simulink model "Linmod_XY_axis_PID_cascade_2021_state_estimator_extra_values"  (R2022b)
settings: Solver=ode4  StartTime=0.0  StopTime=68  FixedStep=1/400  RelTol=1e-3
undefined symbols (not defined in the file): Quad
libraries: simulink x2
settings Model: Creator=laurentburlion  LastModifiedBy=blank
settings ModelReferenceCC: EnableRefExpFcnMdlSchedulingChecks=on

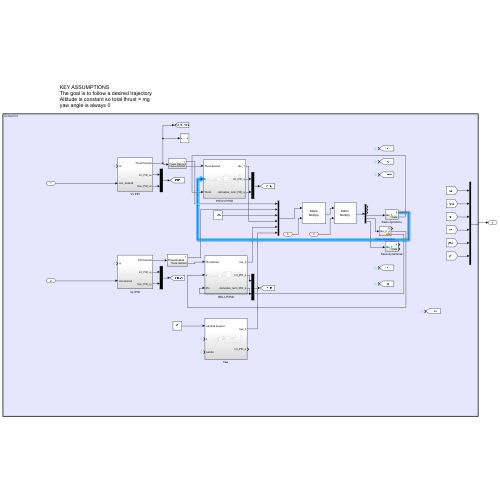
[thumbnail: Simulink's stored preview of the top-level diagram]
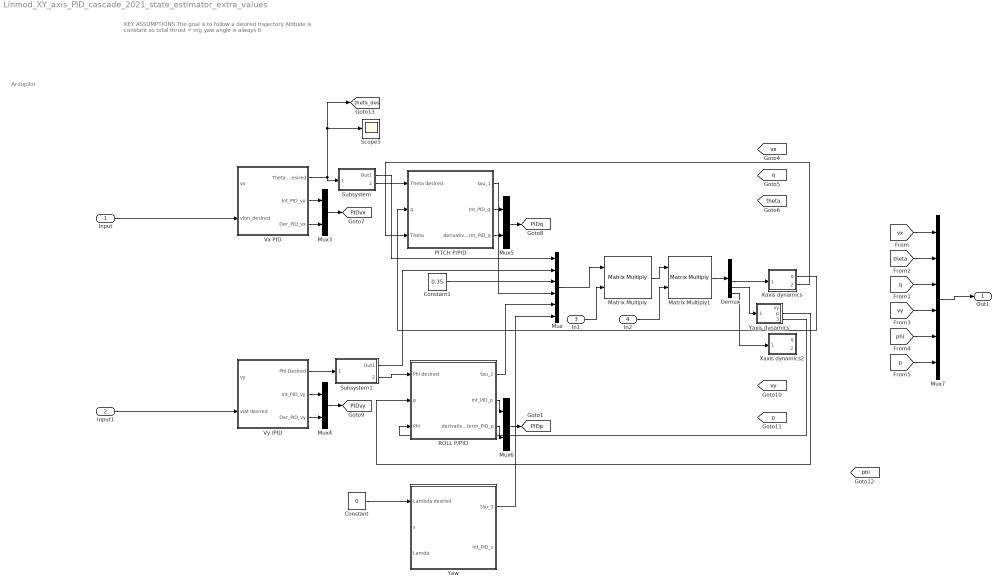
== system Linmod_XY_axis_PID_cascade_2021_state_estimator_extra_values ==
  note: Ardupilot
  note: KEY ASSUMPTIONS
      | The goal is to follow a desired trajectory
      | Altitude is constant so total thrust = mg
      | yaw angle is always 0
  Input : Inport
  Input1 : Inport  Port=2
  In1 : Inport  Port=3
  In2 : Inport  Port=4
  Constant : Constant  Value=0
  Constant1 : Constant  Value=0.35
  Demux : Demux  Outputs=6
  Matrix Multiply : Product  Multiplication=Matrix(*)
  Matrix Multiply1 : Product  Multiplication=Matrix(*)
  Mux : Mux  Inputs=6
  Mux{3..6} (4 alike) : Mux  Inputs=2
  Mux7 : Mux  Inputs=6
  PITCH P/PID : Subsystem
  ROLL P/PID : Subsystem
  Scope5 : Scope
  Subsystem : Subsystem
  Subsystem1 : Subsystem
  Vx PID : Subsystem
  Vy /PID : Subsystem
  Xaxis dynamics : Subsystem
  Xaxis dynamics2 : Subsystem
  "Yaw " : Subsystem
  Yaxis dynamics : Subsystem
  Out1 : Outport
  tag scope: PIDp=global, PIDq=global, PIDvx=global, PIDvy=global, p=global, phi=global, q=global, theta=global, theta_des=global, vx=global, vy=global
  wires:
  Vy /PID/1(Phi Desired) -> Subsystem1/1(Theta Desired)
  Vx PID/1(Theta Desired) -> Subsystem/1(Theta Desired), [theta_des], Scope5/1
  Vy /PID/3(Der_PID_vy) -> Mux4/2
  Vy /PID/2(Int_PID_vy) -> Mux4/1
  Mux4/1 -> [PIDvy]
  Vx PID/2(Int_PID_vx) -> Mux3/1
  Vx PID/3(Der_PID_vx) -> Mux3/2
  Mux3/1 -> [PIDvx]
  PITCH P/PID/3(derivative_term_PID_q) -> Mux5/2
  PITCH P/PID/2(Int_PID_q) -> Mux5/1
  Mux5/1 -> [PIDq]
  ROLL P/PID/2(Int_PID_p) -> Mux6/1
  ROLL P/PID/3(derivative_term_PID_p) -> Mux6/2
  Mux6/1 -> [PIDp]
  Input/1 -> Vx PID/2(vlon_desired)
  Input1/1 -> Vy /PID/2(vlat desired)
  [vx] -> Mux7/1
  [q] -> Mux7/3
  [theta] -> Mux7/2
  [vy] -> Mux7/4
  [p] -> Mux7/6
  [phi] -> Mux7/5
  Mux7/1 -> Out1/1
  Subsystem/2(Theta desired) -> PITCH P/PID/1(Theta desired)
  Subsystem1/2(Theta desired) -> ROLL P/PID/1(Phi desired)
  Constant/1 -> "Yaw "/1(Lambda desired)
  Subsystem/1(Out1) -> Mux/1
  Subsystem1/1(Out1) -> Mux/2
  PITCH P/PID/1(tau_1) -> Mux/4
  ROLL P/PID/1(tau_2) -> Mux/5
  "Yaw "/1(tau_3) -> Mux/6
  Mux/1 -> Matrix Multiply/1
  Constant1/1 -> Mux/3
  In1/1 -> Matrix Multiply/2
  Matrix Multiply/1 -> Matrix Multiply1/1
  In2/1 -> Matrix Multiply1/2
  Matrix Multiply1/1 -> Demux/1
  Demux/4 -> Xaxis dynamics/1(tau_1)
  Demux/5 -> Yaxis dynamics/1(tau_2)
  Demux/6 -> Xaxis dynamics2/1(tau_1)
  Xaxis dynamics/1(q) -> PITCH P/PID/2(q)
  Xaxis dynamics/2(theta) -> PITCH P/PID/3(Theta)
  Yaxis dynamics/2(p) -> ROLL P/PID/2(p)
  Yaxis dynamics/3(phi) -> ROLL P/PID/3(Phi)

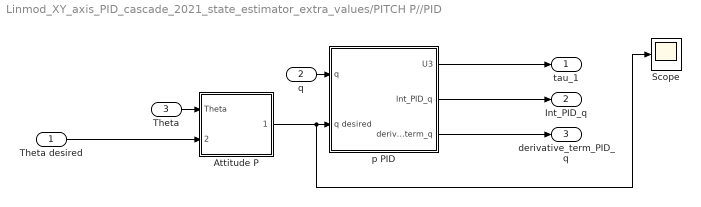
== system Linmod_XY_axis_PID_cascade_2021_state_estimator_extra_values/PITCH P//PID ==
  Theta desired : Inport
  q : Inport  Port=2
  Theta : Inport  Port=3
  Attitude P : Subsystem
  Scope : Scope
  p PID : Subsystem
  tau_1 : Outport
  Int_PID_q : Outport  Port=2
  derivative_term_PID_q : Outport  Port=3
  wires:
  p PID/1(U3) -> tau_1/1
  Attitude P/1(q desired) -> Scope/1, p PID/2(q desired)
  Theta/1 -> Attitude P/1(Theta)
  q/1 -> p PID/1(q)
  Theta desired/1 -> Attitude P/2(Theta desired)
  p PID/2(Int_PID_q) -> Int_PID_q/1
  p PID/3(derivative_term_q) -> derivative_term_PID_q/1

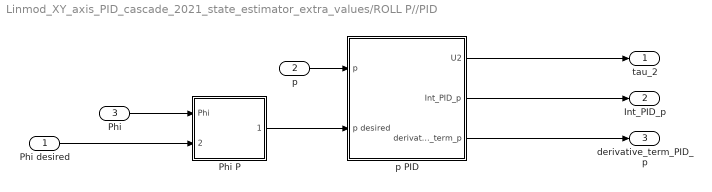
== system Linmod_XY_axis_PID_cascade_2021_state_estimator_extra_values/ROLL P//PID ==
  Phi desired : Inport
  p : Inport  Port=2
  Phi : Inport  Port=3
  Phi P : Subsystem
  p PID : Subsystem
  tau_2 : Outport
  Int_PID_p : Outport  Port=2
  derivative_term_PID_p : Outport  Port=3
  wires:
  Phi desired/1 -> Phi P/2(Phi desired)
  p/1 -> p PID/1(p)
  Phi/1 -> Phi P/1(Phi)
  Phi P/1(p desired) -> p PID/2(p desired)
  p PID/1(U2) -> tau_2/1
  p PID/2(Int_PID_p) -> Int_PID_p/1
  p PID/3(derivative_term_p) -> derivative_term_PID_p/1

== system Linmod_XY_axis_PID_cascade_2021_state_estimator_extra_values/Subsystem ==
  Theta Desired : Inport
  Constant : Constant  Value=0.0
  Sine : simulink/Lookup Tables/Sine  Formula=sin(2*pi*u)  NumDataPoints=(2^5)+1  OutputWordLength=16  InternalRulePriority=Speed
  Out1 : Outport
  Theta desired : Outport  Port=2
  wires:
  Theta Desired/1 -> Sine/1
  Sine/1 -> Out1/1
  Constant/1 -> Theta desired/1

== system Linmod_XY_axis_PID_cascade_2021_state_estimator_extra_values/Subsystem1 ==
  Theta Desired : Inport
  Constant : Constant  Value=0.0
  Cosine : simulink/Lookup Tables/Cosine  Formula=cos(2*pi*u)  NumDataPoints=(2^5)+1  OutputWordLength=16  InternalRulePriority=Speed
  Out1 : Outport
  Theta desired : Outport  Port=2
  wires:
  Theta Desired/1 -> Cosine/1
  Cosine/1 -> Out1/1
  Constant/1 -> Theta desired/1

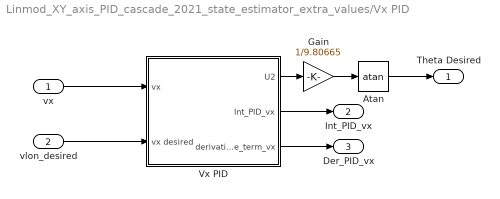
== system Linmod_XY_axis_PID_cascade_2021_state_estimator_extra_values/Vx PID ==
  vx : Inport
  vlon_desired : Inport  Port=2
  Atan : Trigonometry  Operator=atan
  Gain : Gain  Gain=1/9.80665
  Vx PID : Subsystem
  Theta Desired : Outport
  Int_PID_vx : Outport  Port=2
  Der_PID_vx : Outport  Port=3
  wires:
  vlon_desired/1 -> Vx PID/2(vx desired)
  vx/1 -> Vx PID/1(vx)
  Vx PID/2(Int_PID_vx) -> Int_PID_vx/1
  Vx PID/3(derivative_term_vx) -> Der_PID_vx/1
  Vx PID/1(U2) -> Gain/1
  Gain/1 -> Atan/1
  Atan/1 -> Theta Desired/1

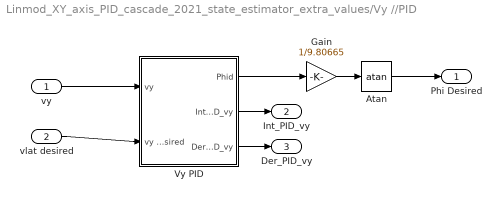
== system Linmod_XY_axis_PID_cascade_2021_state_estimator_extra_values/Vy //PID ==
  vy : Inport
  vlat desired : Inport  Port=2
  Atan : Trigonometry  Operator=atan
  Gain : Gain  Gain=1/9.80665
  Vy PID : Subsystem
  Phi Desired : Outport
  Int_PID_vy : Outport  Port=2
  Der_PID_vy : Outport  Port=3
  wires:
  Vy PID/2(Int_PID_vy) -> Int_PID_vy/1
  vy/1 -> Vy PID/1(vy)
  vlat desired/1 -> Vy PID/2(vy desired)
  Vy PID/3(Derivative_PID_vy) -> Der_PID_vy/1
  Vy PID/1(Phid) -> Gain/1
  Gain/1 -> Atan/1
  Atan/1 -> Phi Desired/1

== system Linmod_XY_axis_PID_cascade_2021_state_estimator_extra_values/Xaxis dynamics ==
  tau_1 : Inport
  Gain : Gain  Gain=1/Quad.Jy
  Integrator : Integrator
  Integrator1 : Integrator
  Scope : Scope
  q : Outport
  theta : Outport  Port=2
  wires:
  Integrator1/1 -> Scope/1, theta/1
  Integrator/1 -> q/1, Integrator1/1
  Gain/1 -> Integrator/1
  tau_1/1 -> Gain/1

== system Linmod_XY_axis_PID_cascade_2021_state_estimator_extra_values/Xaxis dynamics2 ==
  tau_1 : Inport
  Gain : Gain  Gain=1/Quad.Jy
  Integrator : Integrator
  Integrator1 : Integrator
  Scope : Scope
  q : Outport
  theta : Outport  Port=2
  wires:
  Integrator1/1 -> Scope/1, theta/1
  Integrator/1 -> q/1, Integrator1/1
  Gain/1 -> Integrator/1
  tau_1/1 -> Gain/1

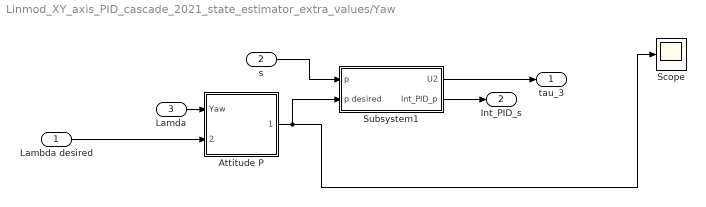
== system Linmod_XY_axis_PID_cascade_2021_state_estimator_extra_values/Yaw  ==
  Lambda desired : Inport
  s : Inport  Port=2
  "Lamda " : Inport  Port=3
  Attitude P : Subsystem
  Scope : Scope
  Subsystem1 : Subsystem
  tau_3 : Outport
  Int_PID_s : Outport  Port=2
  wires:
  s/1 -> Subsystem1/1(p)
  Subsystem1/1(U2) -> tau_3/1
  Subsystem1/2(Int_PID_p) -> Int_PID_s/1
  Attitude P/1(q desired) -> Subsystem1/2(p desired), Scope/1
  Lambda desired/1 -> Attitude P/2(Yaw desired)
  "Lamda "/1 -> Attitude P/1(Yaw)

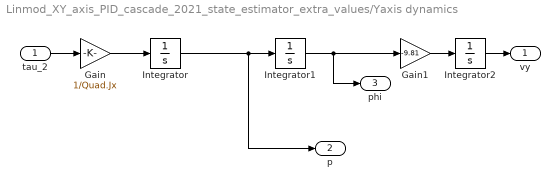
== system Linmod_XY_axis_PID_cascade_2021_state_estimator_extra_values/Yaxis dynamics ==
  tau_2 : Inport
  Gain : Gain  Gain=1/Quad.Jx
  Gain1 : Gain  Gain=-9.81
  Integrator : Integrator
  Integrator1 : Integrator
  Integrator2 : Integrator
  vy : Outport
  p : Outport  Port=2
  phi : Outport  Port=3
  wires:
  tau_2/1 -> Gain/1
  Gain/1 -> Integrator/1
  Integrator/1 -> Integrator1/1, p/1
  Integrator1/1 -> phi/1, Gain1/1
  Gain1/1 -> Integrator2/1
  Integrator2/1 -> vy/1

== system Linmod_XY_axis_PID_cascade_2021_state_estimator_extra_values/PITCH P//PID/Attitude P ==
  Theta : Inport
  Theta desired : Inport  Port=2
  Kp : Gain  Gain=Quad.phi_KP
  Theta Error : Sum  Inputs=+-
  q desired : Outport
  wires:
  Theta Error/1 -> Kp/1
  Kp/1 -> q desired/1
  Theta desired/1 -> Theta Error/1
  Theta/1 -> Theta Error/2

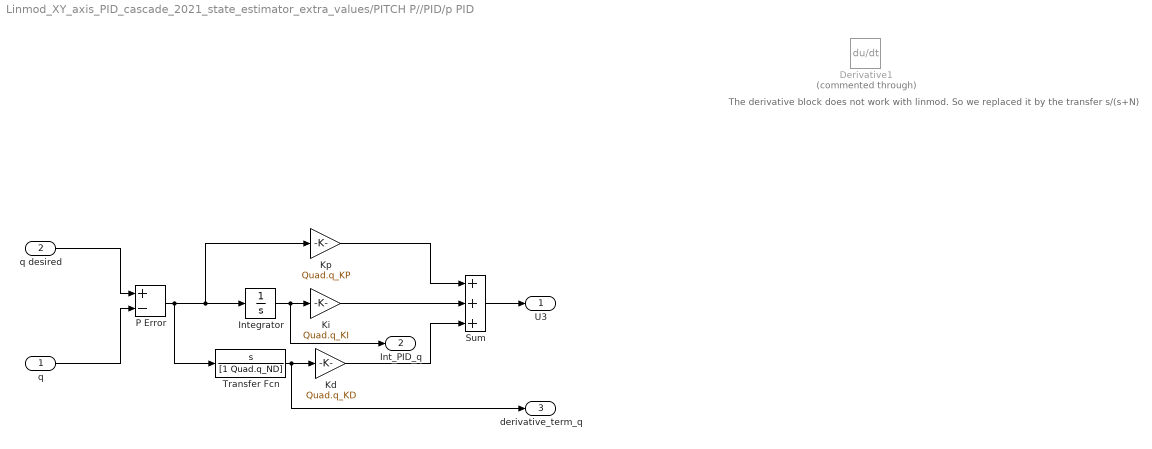
== system Linmod_XY_axis_PID_cascade_2021_state_estimator_extra_values/PITCH P//PID/p PID ==
  note: The derivative block does not work with linmod. So we replaced it by the transfer s/(s+N)
  q : Inport
  q desired : Inport  Port=2
  Derivative1 : Derivative  Commented=through
  Integrator : Integrator
  Kd : Gain  Gain=Quad.q_KD
  Ki : Gain  Gain=Quad.q_KI
  Kp : Gain  Gain=Quad.q_KP
  P Error : Sum  Inputs=+-
  Sum : Sum  Inputs=+++
  Transfer Fcn : TransferFcn  Numerator=[1 0]  Denominator=[1 Quad.q_ND]
  U3 : Outport
  Int_PID_q : Outport  Port=2
  derivative_term_q : Outport  Port=3
  wires:
  Ki/1 -> Sum/2
  Kd/1 -> Sum/3
  Integrator/1 -> Int_PID_q/1, Ki/1
  Sum/1 -> U3/1
  Kp/1 -> Sum/1
  q desired/1 -> P Error/1
  q/1 -> P Error/2
  P Error/1 -> Transfer Fcn/1, Kp/1, Integrator/1
  Transfer Fcn/1 -> derivative_term_q/1, Kd/1

== system Linmod_XY_axis_PID_cascade_2021_state_estimator_extra_values/ROLL P//PID/Phi P ==
  Phi : Inport
  Phi desired : Inport  Port=2
  Kp : Gain  Gain=Quad.phi_KP
  Phi Error : Sum  Inputs=+-
  p desired : Outport
  wires:
  Phi/1 -> Phi Error/2
  Phi desired/1 -> Phi Error/1
  Kp/1 -> p desired/1
  Phi Error/1 -> Kp/1

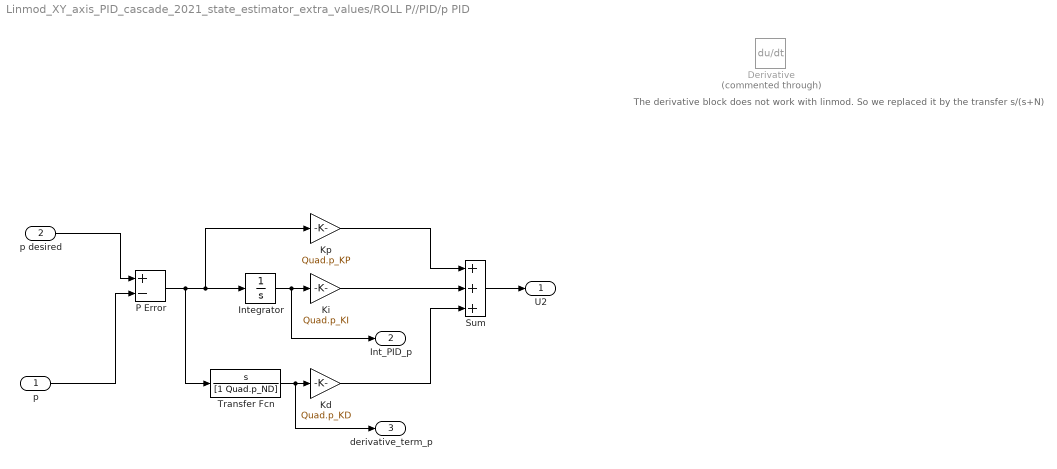
== system Linmod_XY_axis_PID_cascade_2021_state_estimator_extra_values/ROLL P//PID/p PID ==
  note: The derivative block does not work with linmod. So we replaced it by the transfer s/(s+N)
  p : Inport
  p desired : Inport  Port=2
  Derivative : Derivative  Commented=through
  Integrator : Integrator
  Kd : Gain  Gain=Quad.p_KD
  Ki : Gain  Gain=Quad.p_KI
  Kp : Gain  Gain=Quad.p_KP
  P Error : Sum  Inputs=+-
  Sum : Sum  Inputs=+++
  Transfer Fcn : TransferFcn  Numerator=[1 0]  Denominator=[1 Quad.p_ND]
  U2 : Outport
  Int_PID_p : Outport  Port=2
  derivative_term_p : Outport  Port=3
  wires:
  p/1 -> P Error/2
  p desired/1 -> P Error/1
  Kp/1 -> Sum/1
  Sum/1 -> U2/1
  Integrator/1 -> Int_PID_p/1, Ki/1
  Kd/1 -> Sum/3
  Ki/1 -> Sum/2
  P Error/1 -> Transfer Fcn/1, Integrator/1, Kp/1
  Transfer Fcn/1 -> derivative_term_p/1, Kd/1

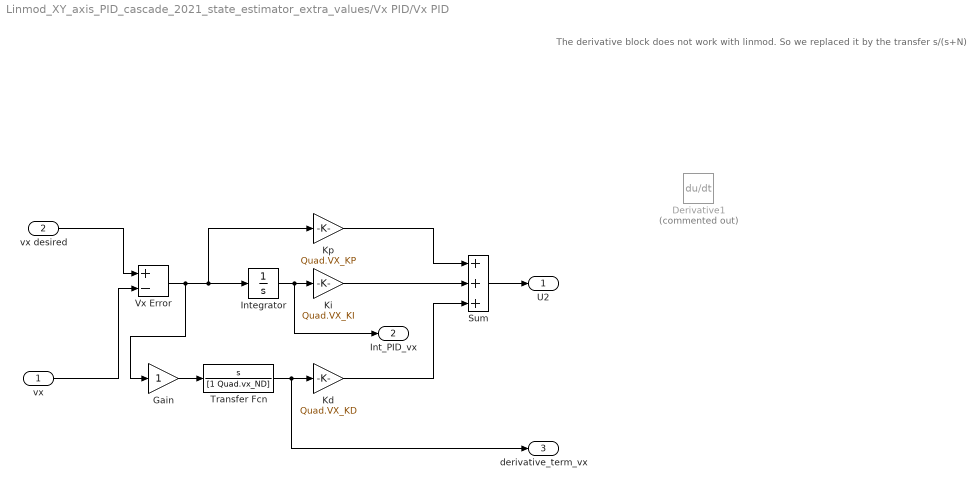
== system Linmod_XY_axis_PID_cascade_2021_state_estimator_extra_values/Vx PID/Vx PID ==
  note: The derivative block does not work with linmod. So we replaced it by the transfer s/(s+N)
  vx : Inport
  vx desired : Inport  Port=2
  Derivative1 : Derivative  Commented=on
  Gain : Gain
  Integrator : Integrator
  Kd : Gain  Gain=Quad.VX_KD
  Ki : Gain  Gain=Quad.VX_KI
  Kp : Gain  Gain=Quad.VX_KP
  Sum : Sum  Inputs=+++
  Transfer Fcn : TransferFcn  Numerator=[1 0]  Denominator=[1 Quad.vx_ND]
  Vx Error : Sum  Inputs=+-
  U2 : Outport
  Int_PID_vx : Outport  Port=2
  derivative_term_vx : Outport  Port=3
  wires:
  vx/1 -> Vx Error/2
  vx desired/1 -> Vx Error/1
  Kp/1 -> Sum/1
  Sum/1 -> U2/1
  Vx Error/1 -> Gain/1, Integrator/1, Kp/1
  Integrator/1 -> Int_PID_vx/1, Ki/1
  Kd/1 -> Sum/3
  Gain/1 -> Transfer Fcn/1
  Ki/1 -> Sum/2
  Transfer Fcn/1 -> derivative_term_vx/1, Kd/1

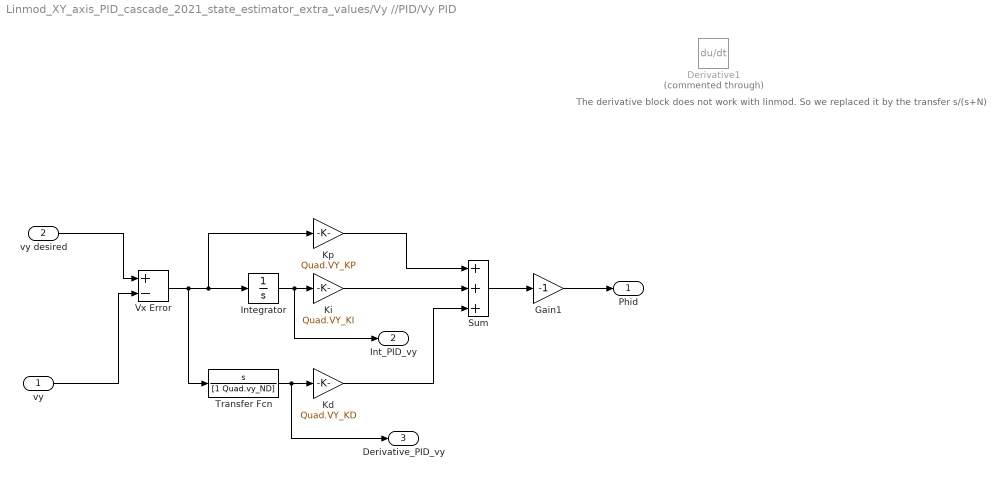
== system Linmod_XY_axis_PID_cascade_2021_state_estimator_extra_values/Vy //PID/Vy PID ==
  note: The derivative block does not work with linmod. So we replaced it by the transfer s/(s+N)
  vy : Inport
  vy desired : Inport  Port=2
  Derivative1 : Derivative  Commented=through
  Gain1 : Gain  Gain=-1
  Integrator : Integrator
  Kd : Gain  Gain=Quad.VY_KD
  Ki : Gain  Gain=Quad.VY_KI
  Kp : Gain  Gain=Quad.VY_KP
  Sum : Sum  Inputs=+++
  Transfer Fcn : TransferFcn  Numerator=[1 0]  Denominator=[1 Quad.vy_ND]
  Vx Error : Sum  Inputs=+-
  Phid : Outport
  Int_PID_vy : Outport  Port=2
  Derivative_PID_vy : Outport  Port=3
  wires:
  Ki/1 -> Sum/2
  Kd/1 -> Sum/3
  Integrator/1 -> Ki/1, Int_PID_vy/1
  Vx Error/1 -> Transfer Fcn/1, Kp/1, Integrator/1
  Sum/1 -> Gain1/1
  Kp/1 -> Sum/1
  vy desired/1 -> Vx Error/1
  vy/1 -> Vx Error/2
  Transfer Fcn/1 -> Derivative_PID_vy/1, Kd/1
  Gain1/1 -> Phid/1

== system Linmod_XY_axis_PID_cascade_2021_state_estimator_extra_values/Yaw /Attitude P ==
  Yaw : Inport
  Yaw desired : Inport  Port=2
  Kp : Gain  Gain=Quad.phi_KP
  Yaw Error : Sum  Inputs=+-
  q desired : Outport
  wires:
  Yaw Error/1 -> Kp/1
  Kp/1 -> q desired/1
  Yaw desired/1 -> Yaw Error/1
  Yaw/1 -> Yaw Error/2

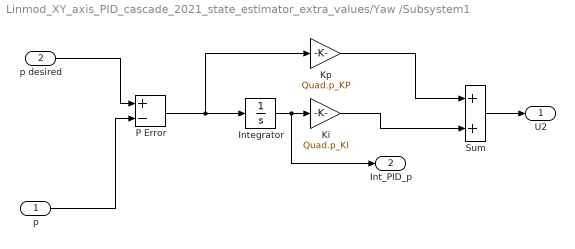
== system Linmod_XY_axis_PID_cascade_2021_state_estimator_extra_values/Yaw /Subsystem1 ==
  p : Inport
  p desired : Inport  Port=2
  Integrator : Integrator
  Ki : Gain  Gain=Quad.p_KI
  Kp : Gain  Gain=Quad.p_KP
  P Error : Sum  Inputs=+-
  Sum : Sum
  U2 : Outport
  Int_PID_p : Outport  Port=2
  wires:
  p desired/1 -> P Error/1
  Ki/1 -> Sum/2
  P Error/1 -> Integrator/1, Kp/1
  Kp/1 -> Sum/1
  p/1 -> P Error/2
  Sum/1 -> U2/1
  Integrator/1 -> Int_PID_p/1, Ki/1
